simulink model "task8_lab14"  (R2021a)
settings: Solver=FixedStepAuto  StartTime=0.0  StopTime=10.0  FixedStep=0.01  RelTol=1e-3
libraries: simulink x1
settings Model: Creator=reemb  LastModifiedBy=reemb

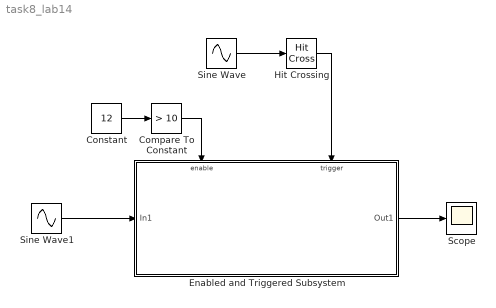
== system task8_lab14 ==
  Compare To Constant : simulink/Logic and Bit Operations/Compare To Constant  relop=>  const=10  OutDataTypeStr=boolean
  Constant : Constant  Value=12
  Enabled and Triggered Subsystem : Subsystem  TreatAsAtomicUnit=on
  Hit Crossing : HitCross
  Scope : Scope
  Sine Wave : Sin  SampleTime=0
  Sine Wave1 : Sin  SampleTime=0
  wires:
  Constant/1 -> Compare To Constant/1
  Compare To Constant/1 -> Enabled and Triggered Subsystem/Enable
  Sine Wave/1 -> Hit Crossing/1
  Hit Crossing/1 -> Enabled and Triggered Subsystem/Trigger
  Enabled and Triggered Subsystem/1(Out1) -> Scope/1
  Sine Wave1/1 -> Enabled and Triggered Subsystem/1(In1)

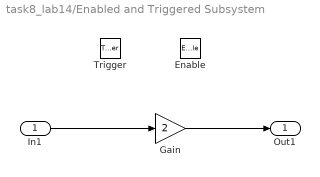
== system task8_lab14/Enabled and Triggered Subsystem ==
  In1 : Inport
  Enable : EnablePort
  Trigger : TriggerPort  VariantControl=(inherit)
  Gain : Gain  Gain=2
  Out1 : Outport
  wires:
  Gain/1 -> Out1/1
  In1/1 -> Gain/1
